simulink model "parameter_id"  (R2014b)
settings: Solver=FixedStepDiscrete  StartTime=0.0  StopTime=inf  FixedStep=sample_time  RelTol=1e-3
undefined symbols (not defined in the file): control_start_time, enable_back_left, enable_back_right, enable_front_left, enable_front_right, g, kd_motor, kp_motor, suspended_mass
libraries: simulink x1
settings Model: xpc_rtwmakecfg_data=_xpcethercatlib_  BufferReuse=off  Creator=wmartin  LastModifiedBy=wmartin
settings SolverCC: EnableConcurrentExecution=on
settings DataIOCC: MaxDataPoints=1000000000  SaveFormat=StructureWithTime
settings OptimizationCC: BlockReduction=off  OptimizeBlockIOStorage=off  BufferReuse=off  GlobalBufferReuse=off  ExpressionFolding=off  ExpressionDepthLimit=2147483647  LocalBlockOutputs=off  SimCompilerOptimization=On
settings DebuggingCC: UnderspecifiedInitializationDetection=Classic  MergeDetectMultiDrivingBlocksExec=none  StateNameClashWarn=warning
settings HardwareCC: ProdIntDivRoundTo=Zero  ProdEndianess=LittleEndian  ProdLongLongMode=on  ProdHWDeviceType=Generic->32-bit x86 compatible
settings ModelReferenceCC: UpdateModelReferenceTargets=IfOutOfDate  EnableParallelModelReferenceBuilds=on
settings RTWCC: SystemTargetFile=slrt.tlc  TemplateMakefile=slrt_default_tmf  Description=Simulink Real-Time  RTWVerbose=off  ProcessScript=slrt_make_rtw_hook  RTWCompilerOptimization=On
settings CodeAppCC: MaxIdLength=256
settings SimulinkRealTimeCC: GeneratePreprocessorConditionals=Disable all  EnableShiftOperators=on  RL32LogBufSizeModifier=100000000

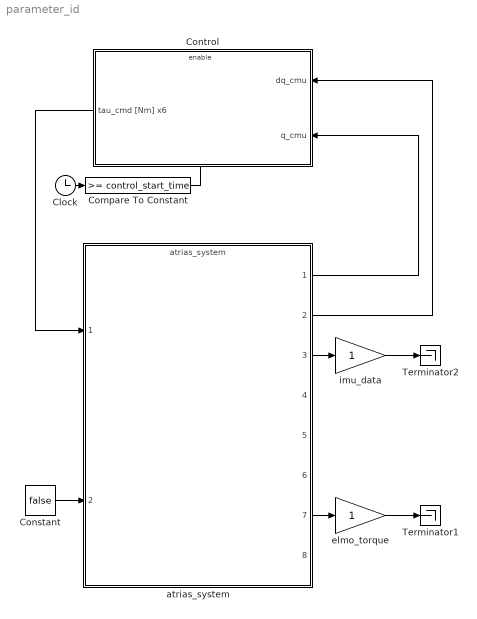
== system parameter_id ==
  Clock : Clock
  Compare To Constant : simulink/Logic and Bit Operations/Compare To Constant  relop=>=  const=control_start_time  OutDataTypeStr=boolean
  Constant : Constant  Value=false
  Control : Subsystem
  Terminator1 : Terminator
  Terminator2 : Terminator
  atrias_system : ModelReference  ModelNameDialog=atrias_system  SimulationMode=Normal  ModelReferenceVersion=1.2649  CopyOfModelName=atrias_system  DefaultDataLogging=on
  elmo_torque : Gain
  imu_data : Gain
  wires:
  Clock/1 -> Compare To Constant/1
  Compare To Constant/1 -> Control/Enable
  atrias_system/1 -> Control/2(q_cmu)
  atrias_system/2 -> Control/1(dq_cmu)
  Constant/1 -> atrias_system/2
  Control/1(tau_cmd [Nm] x6) -> atrias_system/1
  imu_data/1 -> Terminator2/1
  atrias_system/3 -> imu_data/1
  atrias_system/7 -> elmo_torque/1
  elmo_torque/1 -> Terminator1/1

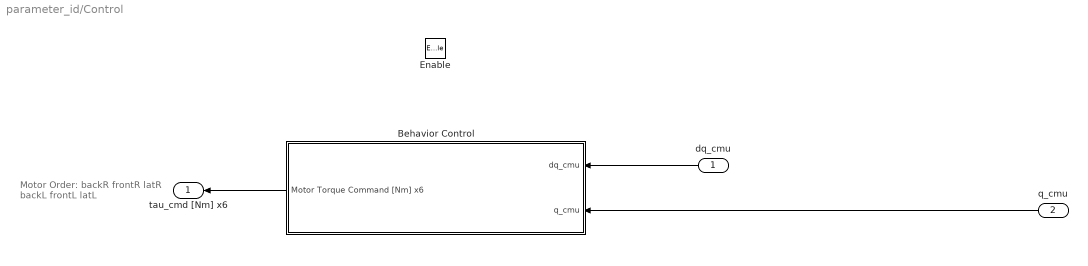
== system parameter_id/Control ==
  note: Motor Order:
      |
      | backR
      | frontR
      | latR
      | backL
      | frontL
      | latL
  dq_cmu : Inport
  q_cmu : Inport  Port=2
  Enable : EnablePort  StatesWhenEnabling=reset
  Behavior Control : Subsystem
  tau_cmd [Nm] x6 : Outport  InitialOutput=[0 0 0 0 0 0]
  wires:
  q_cmu/1 -> Behavior Control/2(q_cmu)
  dq_cmu/1 -> Behavior Control/1(dq_cmu)
  Behavior Control/1(Motor Torque Command [Nm] x6) -> tau_cmd [Nm] x6/1

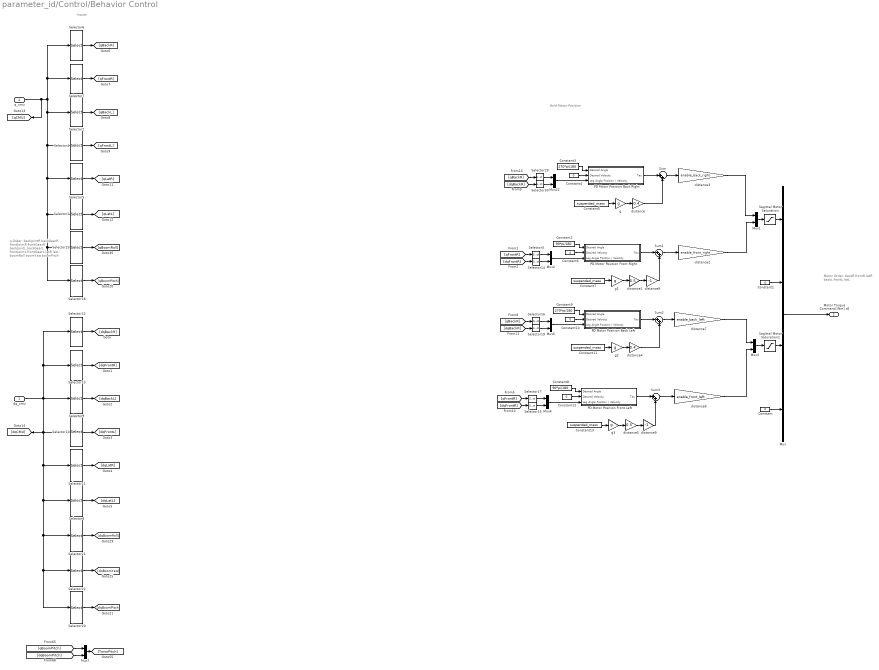
== system parameter_id/Control/Behavior Control ==
  note: Hold Motor Position
  note: Inputs
  note: q Order:
      |
      | backJointR
      | backGearR
      | frontJointR
      | frontGearR
      |
      | backJointL
      | backGearL
      | frontJointL
      | frontGearL
      |
      | latR
      | latL
      |
      | boomRoll
      | boomYaw
      | boomPitch
  note: Motor Order:
      |
      | backR
      | frontR
      | latR
      | backL
      | frontL
      | latL
  dq_cmu : Inport
  q_cmu : Inport  Port=2
  Constant{,1,4,6,10,12} (6 alike) : Constant  Value=0
  Constant{5,7,11,13} (4 alike) : Constant  Value=suspended_mass
  Constant2 : Constant  Value=90*pi/180
  Constant3 : Constant  Value=270*pi/180
  Constant8 : Constant  Value=90*pi/180
  Constant9 : Constant  Value=270*pi/180
  Mux : Mux
  Mux{1..5,7,22} (7 alike) : Mux  Inputs=2
  PD Motor Position Back Left : Subsystem
  PD Motor Position Back Right : Subsystem
  PD Motor Position Front Left : Subsystem
  PD Motor Position Front Right : Subsystem
  Sagittal Motor Saturation : Saturate  UpperLimit=595  LowerLimit=-595
      settings: AttributesFormatString=Top: %<UpperLimit>\nBottom: %<LowerLimit>
  Sagittal Motor Saturation1 : Saturate  UpperLimit=595  LowerLimit=-595
      settings: AttributesFormatString=Top: %<UpperLimit>\nBottom: %<LowerLimit>
  Selector1 : Selector  InputPortWidth=13  Indices=[10]
  Selector10 : Selector  InputPortWidth=13  Indices=[7 8]
  Selector11 : Selector  InputPortWidth=13  Indices=[9]
  Selector12 : Selector  InputPortWidth=13  Indices=[1 2]
  Selector13 : Selector  InputPortWidth=13  Indices=[3 4]
  Selector{3,14..17,19,29..30} (8 alike) : Selector  InputPortWidth=2  Indices=[1]
  Selector18 : Selector  InputPortWidth=13  Indices=[13]
  Selector2 : Selector  InputPortWidth=13  Indices=[5 6]
  Selector20 : Selector  InputPortWidth=13  Indices=[13]
  Selector21 : Selector  InputPortWidth=13  Indices=[11]
  Selector22 : Selector  InputPortWidth=13  Indices=[12]
  Selector23 : Selector  InputPortWidth=13  Indices=[11]
  Selector4 : Selector  InputPortWidth=13  Indices=[7 8]
  Selector5 : Selector  InputPortWidth=13  Indices=[9]
  Selector6 : Selector  InputPortWidth=13  Indices=[1 2]
  Selector7 : Selector  InputPortWidth=13  Indices=[3 4]
  Selector8 : Selector  InputPortWidth=13  Indices=[10]
  Selector9 : Selector  InputPortWidth=13  Indices=[5 6]
  Sum{,1..3} (4 alike) : Sum  Inputs=|++
  distance : Gain  Gain=0.4
  distance1 : Gain  Gain=0.5
  distance2 : Gain  Gain=enable_front_right
  distance3 : Gain  Gain=enable_back_right
  distance4 : Gain  Gain=0.4
  distance5 : Gain  Gain=0.5
  distance6 : Gain  Gain=enable_front_left
  distance7 : Gain  Gain=enable_back_left
  distance8 : Gain  Gain=-1
  distance9 : Gain  Gain=-1
  g{,1..3} (4 alike) : Gain  Gain=g
  Motor Torque Command [Nm] x6 : Outport  OutputWhenDisabled=reset  InitialOutput=[0 0 0 0 0 0]
  wires:
  Constant/1 -> Mux/4
  Constant1/1 -> Mux/2
  Mux7/1 -> [TorsoPitch]
  [dqBoomPitch] -> Mux7/2
  [qBoomPitch] -> Mux7/1
  Selector23/1 -> [qBoomRoll]
  Selector21/1 -> [dqBoomRoll]
  dq_cmu/1 -> Selector9/1, Selector13/1, Selector12/1, [dqCMU], Selector10/1, Selector11/1, Selector8/1, Selector21/1, Selector22/1, Selector20/1
  Selector22/1 -> [dqBoomYaw]
  Selector20/1 -> [dqBoomPitch]
  Selector18/1 -> [qBoomPitch]
  q_cmu/1 -> [qCMU], Selector1/1, Selector23/1, Selector18/1, Selector5/1, Selector4/1, Selector2/1, Selector7/1, Selector6/1
  Selector10/1 -> [dqFrontL]
  Selector9/1 -> [dqBackL]
  Selector13/1 -> [dqFrontR]
  Selector12/1 -> [dqBackR]
  Selector11/1 -> [dqLatR]
  Selector8/1 -> [dqLatL]
  Mux/1 -> Motor Torque Command [Nm] x6/1
  Selector5/1 -> [qLatR]
  Selector1/1 -> [qLatL]
  Selector6/1 -> [qBackR]
  Selector7/1 -> [qFrontR]
  Selector2/1 -> [qBackL]
  Selector4/1 -> [qFrontL]
  PD Motor Position Back Right/1(Tau) -> Sum/1
  Selector29/1 -> Mux22/1
  Selector30/1 -> Mux22/2
  Mux22/1 -> PD Motor Position Back Right/3(Leg Angle Position / Velocity)
  [dqBackR] -> Selector30/1
  [qBackR] -> Selector29/1
  Sum1/1 -> distance2/1
  Mux1/1 -> Sagittal Motor Saturation/1
  Constant4/1 -> PD Motor Position Back Right/2(Desired Velocity)
  Constant3/1 -> PD Motor Position Back Right/1(Desired Angle)
  Sum/1 -> distance3/1
  Constant5/1 -> g/1
  distance/1 -> Sum/2
  g/1 -> distance/1
  PD Motor Position Front Right/1(Tau) -> Sum1/1
  Selector3/1 -> Mux2/1
  Selector14/1 -> Mux2/2
  Mux2/1 -> PD Motor Position Front Right/3(Leg Angle Position / Velocity)
  [dqFrontR] -> Selector14/1
  [qFrontR] -> Selector3/1
  Constant6/1 -> PD Motor Position Front Right/2(Desired Velocity)
  Constant2/1 -> PD Motor Position Front Right/1(Desired Angle)
  Constant7/1 -> g1/1
  distance1/1 -> distance8/1
  g1/1 -> distance1/1
  distance2/1 -> Mux1/2
  distance3/1 -> Mux1/1
  Mux3/1 -> Sagittal Motor Saturation1/1
  PD Motor Position Back Left/1(Tau) -> Sum2/1
  Selector16/1 -> Mux5/1
  Selector19/1 -> Mux5/2
  Mux5/1 -> PD Motor Position Back Left/3(Leg Angle Position / Velocity)
  [dqBackR] -> Selector19/1
  [qBackR] -> Selector16/1
  Sum3/1 -> distance6/1
  Constant10/1 -> PD Motor Position Back Left/2(Desired Velocity)
  Constant9/1 -> PD Motor Position Back Left/1(Desired Angle)
  Sum2/1 -> distance7/1
  Constant11/1 -> g2/1
  distance4/1 -> Sum2/2
  g2/1 -> distance4/1
  PD Motor Position Front Left/1(Tau) -> Sum3/1
  Selector17/1 -> Mux4/1
  Selector15/1 -> Mux4/2
  Mux4/1 -> PD Motor Position Front Left/3(Leg Angle Position / Velocity)
  [dqFrontR] -> Selector15/1
  [qFrontR] -> Selector17/1
  Constant12/1 -> PD Motor Position Front Left/2(Desired Velocity)
  Constant8/1 -> PD Motor Position Front Left/1(Desired Angle)
  Constant13/1 -> g3/1
  distance5/1 -> distance9/1
  g3/1 -> distance5/1
  distance7/1 -> Mux3/1
  distance6/1 -> Mux3/2
  distance8/1 -> Sum1/2
  distance9/1 -> Sum3/2
  Sagittal Motor Saturation/1 -> Mux/1
  Sagittal Motor Saturation1/1 -> Mux/3

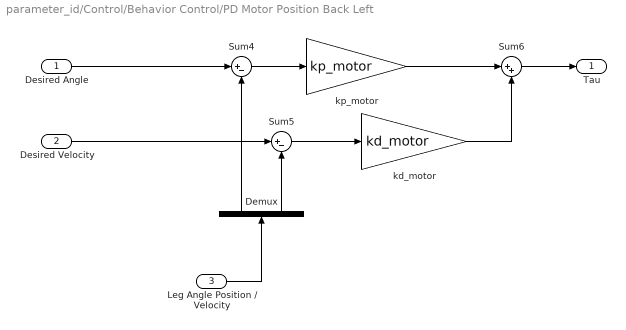
== system parameter_id/Control/Behavior Control/PD Motor Position Back Left ==
  Desired Angle : Inport
  Desired Velocity : Inport  Port=2
  Leg Angle Position / Velocity : Inport  Port=3
  Demux : Demux  Outputs=2
  Sum4 : Sum  Inputs=|+-
  Sum5 : Sum  Inputs=|+-
  Sum6 : Sum  Inputs=|++
  kd_motor : Gain  Gain=kd_motor
  kp_motor : Gain  Gain=kp_motor
  Tau : Outport
  wires:
  Sum6/1 -> Tau/1
  Desired Angle/1 -> Sum4/1
  Demux/1 -> Sum4/2
  Leg Angle Position / Velocity/1 -> Demux/1
  Desired Velocity/1 -> Sum5/1
  Sum4/1 -> kp_motor/1
  Sum5/1 -> kd_motor/1
  kp_motor/1 -> Sum6/1
  Demux/2 -> Sum5/2
  kd_motor/1 -> Sum6/2

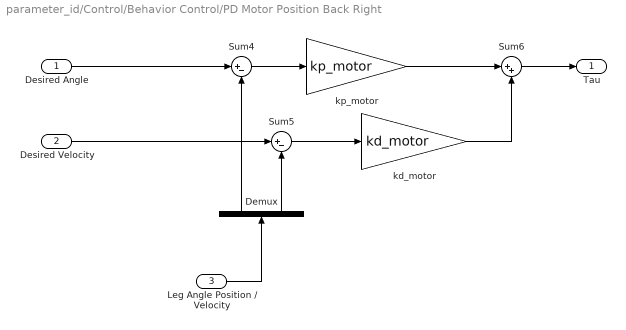
== system parameter_id/Control/Behavior Control/PD Motor Position Back Right ==
  Desired Angle : Inport
  Desired Velocity : Inport  Port=2
  Leg Angle Position / Velocity : Inport  Port=3
  Demux : Demux  Outputs=2
  Sum4 : Sum  Inputs=|+-
  Sum5 : Sum  Inputs=|+-
  Sum6 : Sum  Inputs=|++
  kd_motor : Gain  Gain=kd_motor
  kp_motor : Gain  Gain=kp_motor
  Tau : Outport
  wires:
  kd_motor/1 -> Sum6/2
  Demux/2 -> Sum5/2
  kp_motor/1 -> Sum6/1
  Sum5/1 -> kd_motor/1
  Sum4/1 -> kp_motor/1
  Desired Velocity/1 -> Sum5/1
  Leg Angle Position / Velocity/1 -> Demux/1
  Demux/1 -> Sum4/2
  Desired Angle/1 -> Sum4/1
  Sum6/1 -> Tau/1

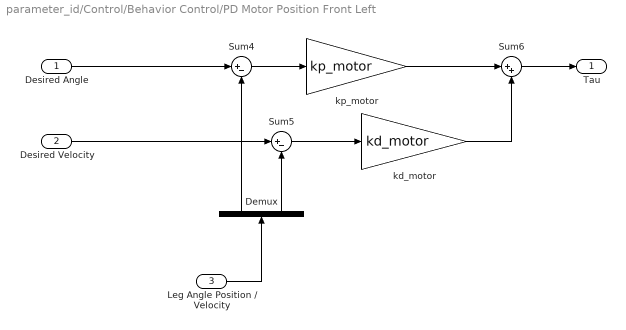
== system parameter_id/Control/Behavior Control/PD Motor Position Front Left ==
  Desired Angle : Inport
  Desired Velocity : Inport  Port=2
  Leg Angle Position / Velocity : Inport  Port=3
  Demux : Demux  Outputs=2
  Sum4 : Sum  Inputs=|+-
  Sum5 : Sum  Inputs=|+-
  Sum6 : Sum  Inputs=|++
  kd_motor : Gain  Gain=kd_motor
  kp_motor : Gain  Gain=kp_motor
  Tau : Outport
  wires:
  kd_motor/1 -> Sum6/2
  Demux/2 -> Sum5/2
  kp_motor/1 -> Sum6/1
  Sum5/1 -> kd_motor/1
  Sum4/1 -> kp_motor/1
  Desired Velocity/1 -> Sum5/1
  Leg Angle Position / Velocity/1 -> Demux/1
  Demux/1 -> Sum4/2
  Desired Angle/1 -> Sum4/1
  Sum6/1 -> Tau/1

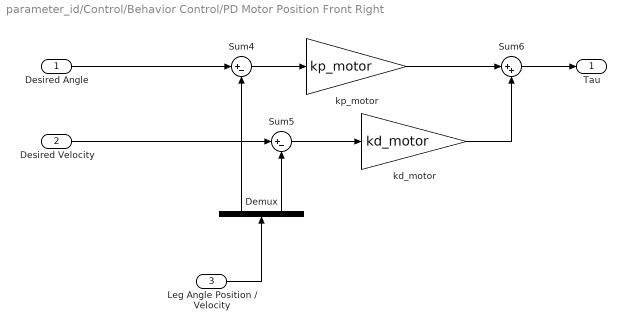
== system parameter_id/Control/Behavior Control/PD Motor Position Front Right ==
  Desired Angle : Inport
  Desired Velocity : Inport  Port=2
  Leg Angle Position / Velocity : Inport  Port=3
  Demux : Demux  Outputs=2
  Sum4 : Sum  Inputs=|+-
  Sum5 : Sum  Inputs=|+-
  Sum6 : Sum  Inputs=|++
  kd_motor : Gain  Gain=kd_motor
  kp_motor : Gain  Gain=kp_motor
  Tau : Outport
  wires:
  Sum6/1 -> Tau/1
  Desired Angle/1 -> Sum4/1
  Demux/1 -> Sum4/2
  Leg Angle Position / Velocity/1 -> Demux/1
  Desired Velocity/1 -> Sum5/1
  Sum4/1 -> kp_motor/1
  Sum5/1 -> kd_motor/1
  kp_motor/1 -> Sum6/1
  Demux/2 -> Sum5/2
  kd_motor/1 -> Sum6/2
